simulink model "IKS02A1_LP_Accel"  (R2024b)
settings: Solver=FixedStepDiscrete  StartTime=0.0  StopTime=inf  RelTol=1e-3  EnableMultiTasking=on
InitFcn:
  | addpath(genpath(pwd));
  | auto_program("IKS02A1_LP_Accel")
  | STLINK_COMPORT = auto_COMPORT()
  | 
  | dialogPrms = get_param(gcs+"/IIS2DLPC", 'DialogParameters');
  | dialogPrmNames = fieldnames(dialogPrms);
  | odr3 = get_param(gcs+"/IIS2DLPC", dialogPrmNames{2});
  | odr3 = eval(odr3);
  | 
  | STM32_ODR = odr3
  | clearvars -except STLINK_COMPORT STLINK_DRIVE STM32_ODR
libraries: etargetslib x5, instrumentseriallib x3
settings Model: SimulationMode=accelerator  PacingRate=1600  ExtModeTrigDuration=10  Creator=JesseJabezArendse  LastModifiedBy=JesseJabezArendse
settings OptimizationCC: ReuseModelBlockBuffer=off  PassReuseOutputArgsAs=Individual arguments  ZeroExternalMemoryAtStartup=off  ZeroInternalMemoryAtStartup=off  MaxStackSize=64  OptimizationLevel=level1  OptimizationCustomize=off  EfficientTunableParamExpr=on
settings DebuggingCC: ParameterPrecisionLossMsg=none  ParameterTunabilityLossMsg=error
settings HardwareCC: ProdHWDeviceType=AMD->x86-64 (Windows64)
settings ModelReferenceCC: EnableParallelModelReferenceBuilds=on
settings SFSimCC: SimParseCustomCode=off  MATLABDynamicMemAlloc=off  SimHardwareAcceleration=native
settings RTWCC: Description=Embedded Coder  SystemTargetFile=ert.tlc  TemplateMakefile=ert_default_tmf  RTWUseSimCustomCode=on  Toolchain=MinGW64 | gmake (64-bit Windows)  BuildConfiguration=Specify  GPUComputeCapability=3.5
settings CodeAppCC: ForceParamTrailComments=on  IgnoreCustomStorageClasses=off  OperatorAnnotations=on  SimulinkDataObjDesc=on  SFDataObjDesc=on  InsertBlockDesc=on
settings ERTTargetCC: CodeReplacementLibrary=GNU C99 extensions  SupportContinuousTime=on  InstructionSetFMA=on  ExtModeTransport=3  ExtModeStaticAlloc=on  ExtModeStaticAllocSize=2000  ExtModeMexFile=ext_xcp  ExtModeIntrfLevel=Level2 - Open  InlinedParameterPlacement=Hierarchical  ERTCustomFileTemplate=example_file_process.tlc  DynamicArrayContainerType=coder::array

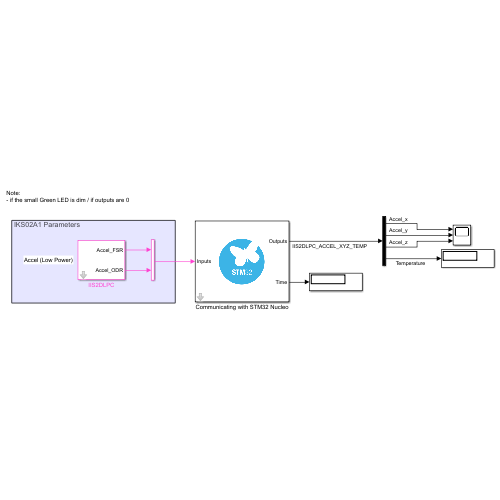
[thumbnail: Simulink's stored preview of the top-level diagram]
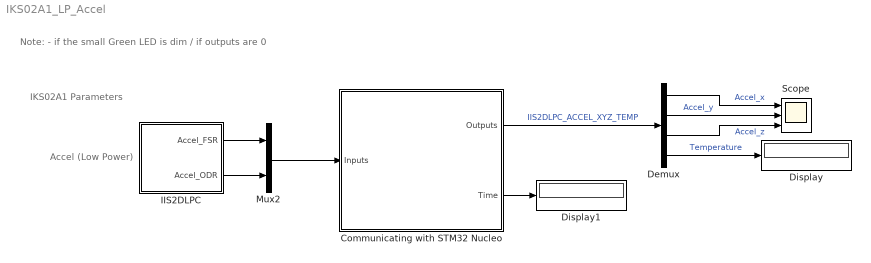
== system IKS02A1_LP_Accel ==
  note: Note:
      | - if the small Green LED is dim / if outputs are 0
  note: IKS02A1 Parameters
  note: Accel (Low Power)
  Communicating with STM32 Nucleo : Subsystem
      mask DialogControl Control1 Prompt: Block for communication between host machine and STM32 Nucleo F411RE
      mask Display: image('stm32_mask_icon.png', [0,0,0,0,80,80]);
  Demux : Demux
  Display : Display
  Display1 : Display
  IIS2DLPC : Subsystem  mask{FSR_AccelOption=16, ODR_AccelOption=200}
      mask prompts: FSR_AccelOption "Full Scale Range (g)"; ODR_AccelOption "Output Data Rate (Hz)"
      mask init:
      | FSR_AccelVals = [2, 4, 8, 16];
      |     FSR_AccelVal = FSR_AccelVals(FSR_AccelOption);
      |     
      |     ODR_AccelVals = [0 , 1.6 , 12.5 , 25 , 50 , 100 , 200 , 400 , 800 , 1600];
      |     ODR_AccelVal = ODR_AccelVals(ODR_AccelOption);
      mask TypeOptions FSR_AccelOption: 2 | 4 | 8 | 16
      mask TypeOptions ODR_AccelOption: 0 | 1.6 | 12.5 | 25 | 50 | 100 | 200 | 400 | 800 | 1600
      mask DialogControl DescGroupVar Prompt: Accelerometer
  Mux2 : Mux  Inputs=2
  Scope : Scope  NumInputPorts=3
  wires:
  Communicating with STM32 Nucleo/1(Outputs) -> Demux/1  "IIS2DLPC_ACCEL_XYZ_TEMP"
  IIS2DLPC/1(Accel_FSR) -> Mux2/1
  IIS2DLPC/2(Accel_ODR) -> Mux2/2
  Mux2/1 -> Communicating with STM32 Nucleo/1(Inputs)
  Communicating with STM32 Nucleo/2(Time) -> Display1/1
  Demux/1 -> Scope/1  "Accel_x"
  Demux/2 -> Scope/2  "Accel_y"
  Demux/3 -> Scope/3  "Accel_z"
  Demux/4 -> Display/1  "Temperature"

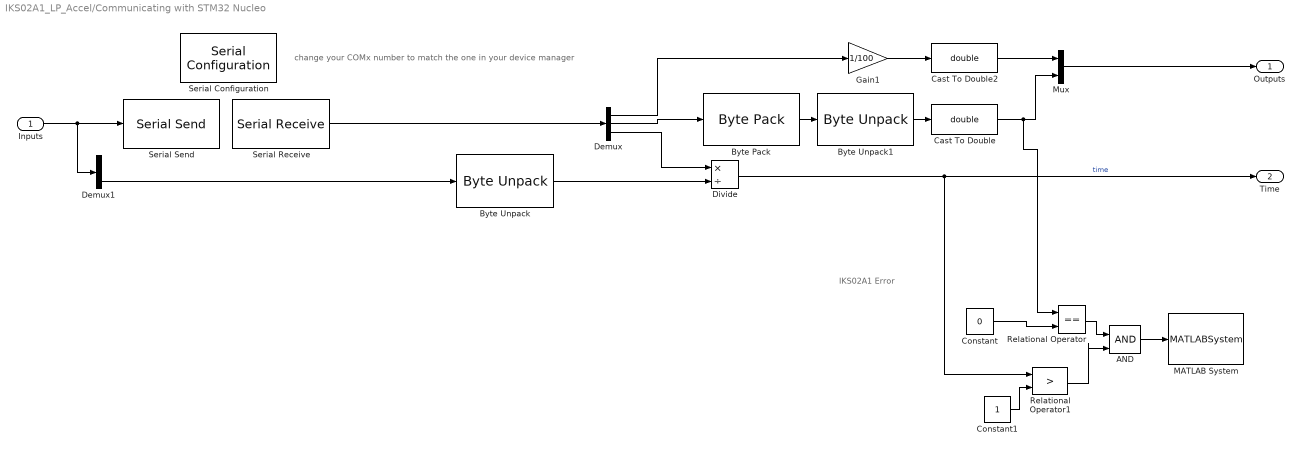
== system IKS02A1_LP_Accel/Communicating with STM32 Nucleo ==
  note: IKS02A1 Error
  note: change your COMx number to match the one in your device manager
  Inputs : Inport
  AND : Logic  IconShape=distinctive  AllPortsSameDT=off  OutDataTypeStr=boolean
  Byte Pack : etargetslib/Byte Pack  datatypes={'int32'}  byteAlign=1
  Byte Unpack : etargetslib/Byte Unpack  dimensions={[1]}  datatypes={'single'}  byteAlign=1
      settings: LibrarySourceBlock=embeddedtargetslib/Host Communication/Byte Unpack
  Byte Unpack1 : etargetslib/Byte Unpack  dimensions={[1]}  datatypes={'single'}  byteAlign=1
      settings: LibrarySourceBlock=embeddedtargetslib/Host Communication/Byte Unpack
  Cast To Double : DataTypeConversion  OutDataTypeStr=double  SaturateOnIntegerOverflow=off  RndMeth=Floor
  Cast To Double2 : DataTypeConversion  OutDataTypeStr=double  SaturateOnIntegerOverflow=off  RndMeth=Floor
  Constant : Constant  Value=0
  Constant1 : Constant
  Demux : Demux  Outputs=[3 1 1]
  Demux1 : Demux  Outputs=[4 4]
  Divide : Product  Inputs=*/
  Gain1 : Gain  Gain=1/100
  MATLAB System : MATLABSystem  System=iks02a1_error  SimulateUsing=Code generation
      mask Type: iks02a1_error
      mask Display:
      | disp('iks02a1_error');
      | port_label('input',1,'u');
  Mux : Mux  Inputs=[3 1]
  Relational Operator : RelationalOperator  Operator===  OutDataTypeStr=boolean  RndMeth=Simplest  InputSameDT=off
  Relational Operator1 : RelationalOperator  Operator=>  OutDataTypeStr=boolean  RndMeth=Simplest  InputSameDT=off
  Serial Configuration : instrumentseriallib/Serial Configuration  Priority=-200000  PortSel=STLINK_COMPORT  Port=STLINK_COMPORT  ComPort=STLINK_COMPORT  BaudRate=1843200  DataBits=8  Parity=even  StopBits=2  ByteOrder=little-endian  FlowControl=none  Timeout=5  SimulateUsing=Interpreted execution  BlockInModel=on  aMode=1
      settings: LibrarySourceBlock=embeddedtargetslib/Host Communication/Serial Configuration
  Serial Receive : instrumentseriallib/Serial Receive  Priority=1  PortSel=STLINK_COMPORT  Port=STLINK_COMPORT  ComPort=STLINK_COMPORT  DataType=int32  SaveDataType=uint8  ToggleHeader=off  Header='J_A'  ToggleDataSize=on  DataSize=[1 5]  ToggleTerminator=on  Terminator=Custom terminator  CustomTerminator='A_J'  InputFormat=Column major  EnableBlockingMode=on  ActionDataUnavailable=Output last received value  ActionWhenDataUnavailable=Output last received value  CustomValue=0  SampleTime=1/STM32_ODR  SimulateUsing=Interpreted execution  BlockInModel=on  aMode=1
      settings: LibrarySourceBlock=embeddedtargetslib/Host Communication/Serial Receive
  Serial Send : instrumentseriallib/Serial Send  Priority=1  PortSel=STLINK_COMPORT  Port=STLINK_COMPORT  ComPort=STLINK_COMPORT  Header='J_A'  Terminator=Custom terminator  CustomTerminator='A_J'  EnableBlockingMode=off  SimulateUsing=Interpreted execution  BlockInModel=on  aMode=1
      settings: LibrarySourceBlock=embeddedtargetslib/Host Communication/Serial Send
  Outputs : Outport
  Time : Outport  Port=2
  wires:
  Inputs/1 -> Demux1/1, Serial Send/1
  Demux/1 -> Gain1/1
  Demux/3 -> Divide/1
  Serial Receive/1 -> Demux/1
  Gain1/1 -> Cast To Double2/1
  Divide/1 -> Time/1, Relational Operator1/1  "time"
  Demux1/2 -> Byte Unpack/1
  Byte Unpack/1 -> Divide/2
  Demux/2 -> Byte Pack/1
  Mux/1 -> Outputs/1
  Byte Pack/1 -> Byte Unpack1/1
  Byte Unpack1/1 -> Cast To Double/1
  Cast To Double/1 -> Relational Operator/1, Mux/2
  Cast To Double2/1 -> Mux/1
  Constant/1 -> Relational Operator/2
  Relational Operator/1 -> AND/1
  AND/1 -> MATLAB System/1
  Relational Operator1/1 -> AND/2
  Constant1/1 -> Relational Operator1/2

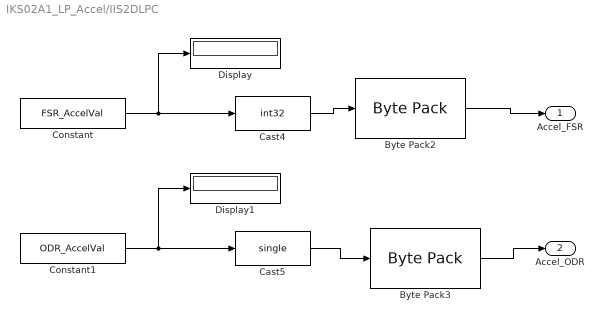
== system IKS02A1_LP_Accel/IIS2DLPC ==
  Byte Pack2 : etargetslib/Byte Pack  datatypes={'int32'}  byteAlign=1
  Byte Pack3 : etargetslib/Byte Pack  datatypes={'single'}  byteAlign=1
  Cast4 : DataTypeConversion  OutDataTypeStr=int32  SaturateOnIntegerOverflow=off  RndMeth=Floor
  Cast5 : DataTypeConversion  OutDataTypeStr=single  SaturateOnIntegerOverflow=off  RndMeth=Floor
  Constant : Constant  Value=FSR_AccelVal
  Constant1 : Constant  Value=ODR_AccelVal
  Display : Display
  Display1 : Display
  Accel_FSR : Outport
  Accel_ODR : Outport  Port=2
  wires:
  Constant/1 -> Cast4/1, Display/1
  Constant1/1 -> Cast5/1, Display1/1
  Cast4/1 -> Byte Pack2/1
  Cast5/1 -> Byte Pack3/1
  Byte Pack2/1 -> Accel_FSR/1
  Byte Pack3/1 -> Accel_ODR/1
